simulink library "hdlmdlgenlib"  (R2019a)
settings: Solver=FixedStepDiscrete  StartTime=0.0  StopTime=10.0  FixedStep=1  RelTol=1e-3  EnableMultiTasking=on
libraries: simulink x25, $bdroot x4
settings Model: Creator=The MathWorks, Inc.  LastModifiedBy=The MathWorks, Inc.
settings DataIOCC: LimitDataPoints=on  SaveFormat=Array  ReturnWorkspaceOutputs=off
settings OptimizationCC: ExpressionDepthLimit=2147483647  LifeSpan=inf
settings DebuggingCC: UnderspecifiedInitializationDetection=Classic  MergeDetectMultiDrivingBlocksExec=none  SolverPrmCheckMsg=warning  FcnCallInpInsideContextMsg=warning  AllowSymbolicDim=off  StateNameClashWarn=warning  PregeneratedLibrarySubsystemCodeDiagnostic=none  SFUnexpectedBacktrackingDiag=warning  SFNoUnconditionalDefaultTransitionDiag=warning  SFExecutionAtInitializationDiag=none  ArithmeticOperatorsInVariantConditions=warning
settings HardwareCC: ProdBitPerPointer=32  ProdBitPerSizeT=32  ProdBitPerPtrDiffT=32  ProdLargestAtomicFloat=None  ProdIntDivRoundTo=Undefined  ProdEndianess=Unspecified  ProdWordSize=32  ProdHWDeviceType=32-bit Generic
settings ModelReferenceCC: PropagateSignalLabelsOutOfModel=off
settings SFSimCC: SimUseLocalCustomCode=off
settings RTWCC: RTWUseLocalCustomCode=off
settings CodeAppCC: StateflowObjectComments=on
settings GRTTargetCC: TargetLangStandard=C89/C90 (ANSI)  GeneratePreprocessorConditionals=Disable all  CombineOutputUpdateFcns=off  GRTInterface=on
settings ConfigComp: CovMetricSettings=dw  CovHtmlReporting=on  CovSaveCumulativeToWorkspaceVar=on  CovSaveSingleToWorkspaceVar=on  CovShowResultsExplorer=off  CovExternalEMLEnable=off

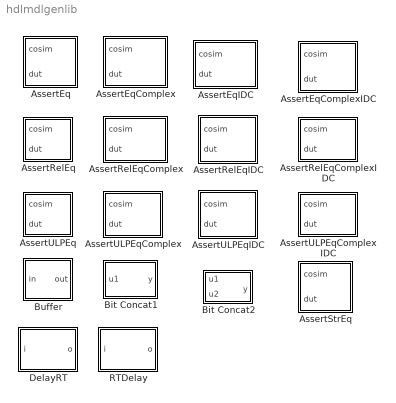
== system hdlmdlgenlib ==
  AssertEq : Subsystem
  AssertEqComplex : Subsystem
  AssertEqComplexIDC : Subsystem
  AssertEqIDC : Subsystem
  AssertRelEq : Subsystem  mask{ToleranceValue=1e-7}
  AssertRelEqComplex : Subsystem  mask{ToleranceValue=1e-7}
  AssertRelEqComplexIDC : Subsystem  mask{ToleranceValue=1e-7}
  AssertRelEqIDC : Subsystem  mask{ToleranceValue=1e-7}
  AssertStrEq : Subsystem  AncestorBlock=hdlmdlgenlib/AssertEq
  AssertULPEq : Subsystem  mask{ToleranceValue=0}
  AssertULPEqComplex : Subsystem  mask{ToleranceValue=0}
  AssertULPEqComplexIDC : Subsystem  mask{ToleranceValue=0}
  AssertULPEqIDC : Subsystem  mask{ToleranceValue=0}
  Bit Concat1 : Subsystem  TreatAsAtomicUnit=on  mask(Bit Concat){}
      mask help: Concatenate the input words.
      mask init:
      | blkname = 'Concat';
      mask Help: helpview([docroot '/toolbox/hdlcoder/ug/hdlcoder_ug.map'],'HDL_bitwise_operator');
      mask Display: disp(blkname);
  Bit Concat2 : Subsystem  TreatAsAtomicUnit=on  mask(Bit Concat){}
      mask help: Concatenate the input words.
      mask init:
      | blkname = 'Concat';
      mask Help: helpview([docroot '/toolbox/hdlcoder/ug/hdlcoder_ug.map'],'HDL_bitwise_operator');
      mask Display: disp(blkname);
  Buffer : Subsystem  mask(Buffer/Wire){}
      mask help: Buffer
  DelayRT : Subsystem
  RTDelay : Subsystem

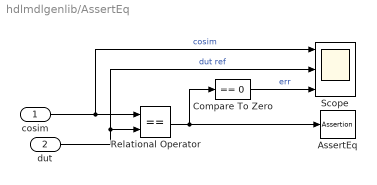
== system hdlmdlgenlib/AssertEq ==
  cosim : Inport
  dut : Inport  Port=2
  AssertEq : Assertion  StopWhenAssertionFail=off
  Compare To Zero : simulink/Logic and Bit Operations/Compare To Zero  relop===  OutDataTypeStr=boolean
  Relational Operator : RelationalOperator  Operator===  OutDataTypeStr=boolean  RndMeth=Nearest
  Scope : Scope  NumInputPorts=3
  wires:
  dut/1 -> Relational Operator/2, Scope/2  "dut ref"
  cosim/1 -> Relational Operator/1, Scope/1  "cosim"
  Relational Operator/1 -> AssertEq/1, Compare To Zero/1
  Compare To Zero/1 -> Scope/3  "err"

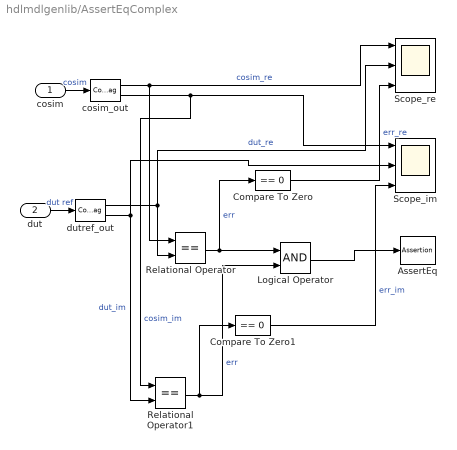
== system hdlmdlgenlib/AssertEqComplex ==
  cosim : Inport
  dut : Inport  Port=2
  AssertEq : Assertion  StopWhenAssertionFail=off
  Compare To Zero : simulink/Logic and Bit Operations/Compare To Zero  relop===  OutDataTypeStr=boolean
  Compare To Zero1 : simulink/Logic and Bit Operations/Compare To Zero  relop===  OutDataTypeStr=boolean
  Logical Operator : Logic  AllPortsSameDT=off  OutDataTypeStr=boolean
  Relational Operator : RelationalOperator  Operator===  OutDataTypeStr=boolean  RndMeth=Nearest
  Relational Operator1 : RelationalOperator  Operator===  OutDataTypeStr=boolean  RndMeth=Nearest
  Scope_im : Scope  NumInputPorts=3
  Scope_re : Scope  NumInputPorts=3
  cosim_out : ComplexToRealImag
  dutref_out : ComplexToRealImag
  wires:
  Relational Operator/1 -> Logical Operator/1, Compare To Zero/1  "err"
  cosim/1 -> cosim_out/1  "cosim"
  dut/1 -> dutref_out/1  "dut ref"
  cosim_out/1 -> Relational Operator/1, Scope_re/1  "cosim_re"
  dutref_out/1 -> Scope_re/2, Relational Operator/2  "dut_re"
  Compare To Zero/1 -> Scope_re/3  "err_re"
  cosim_out/2 -> Relational Operator1/1, Scope_im/1  "cosim_im"
  dutref_out/2 -> Scope_im/2, Relational Operator1/2  "dut_im"
  Compare To Zero1/1 -> Scope_im/3  "err_im"
  Logical Operator/1 -> AssertEq/1
  Relational Operator1/1 -> Logical Operator/2, Compare To Zero1/1  "err"

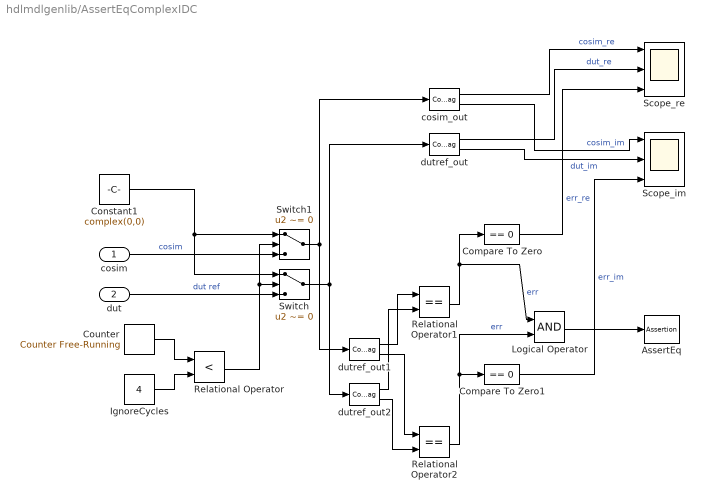
== system hdlmdlgenlib/AssertEqComplexIDC ==
  cosim : Inport
  dut : Inport  Port=2
  AssertEq : Assertion  StopWhenAssertionFail=off
  Compare To Zero : simulink/Logic and Bit Operations/Compare To Zero  relop===  OutDataTypeStr=boolean
  Compare To Zero1 : simulink/Logic and Bit Operations/Compare To Zero  relop===  OutDataTypeStr=boolean
  Constant1 : Constant  Value=complex(0,0)  OutDataTypeStr=Inherit: Inherit via back propagation  SampleTime=-1
  Counter : simulink/Sources/Counter Free-Running  NumBits=32  tsamp=-1
  IgnoreCycles : Constant  Value=4  OutDataTypeStr=Inherit: Inherit via back propagation  SampleTime=-1
  Logical Operator : Logic  AllPortsSameDT=off  OutDataTypeStr=boolean
  Relational Operator : RelationalOperator  Operator=<  OutDataTypeStr=boolean  RndMeth=Nearest
  Relational Operator1 : RelationalOperator  Operator===  OutDataTypeStr=boolean  RndMeth=Nearest
  Relational Operator2 : RelationalOperator  Operator===  OutDataTypeStr=boolean  RndMeth=Nearest
  Scope_im : Scope  NumInputPorts=3
  Scope_re : Scope  NumInputPorts=3
  Switch : Switch  Criteria=u2 ~= 0
  Switch1 : Switch  Criteria=u2 ~= 0
  cosim_out : ComplexToRealImag
  dutref_out : ComplexToRealImag
  dutref_out1 : ComplexToRealImag
  dutref_out2 : ComplexToRealImag
  wires:
  Compare To Zero1/1 -> Scope_im/3  "err_im"
  dutref_out/2 -> Scope_im/2  "dut_im"
  cosim_out/2 -> Scope_im/1  "cosim_im"
  Compare To Zero/1 -> Scope_re/3  "err_re"
  dutref_out/1 -> Scope_re/2  "dut_re"
  cosim_out/1 -> Scope_re/1  "cosim_re"
  Relational Operator1/1 -> Logical Operator/1, Compare To Zero/1  "err"
  Switch1/1 -> dutref_out1/1, cosim_out/1
  Switch/1 -> dutref_out2/1, dutref_out/1
  Constant1/1 -> Switch1/1, Switch/1
  Relational Operator/1 -> Switch1/2, Switch/2
  cosim/1 -> Switch1/3  "cosim"
  dut/1 -> Switch/3  "dut ref"
  Counter/1 -> Relational Operator/1
  IgnoreCycles/1 -> Relational Operator/2
  Logical Operator/1 -> AssertEq/1
  dutref_out1/1 -> Relational Operator1/1
  dutref_out2/1 -> Relational Operator1/2
  dutref_out2/2 -> Relational Operator2/2
  dutref_out1/2 -> Relational Operator2/1
  Relational Operator2/1 -> Logical Operator/2, Compare To Zero1/1  "err"

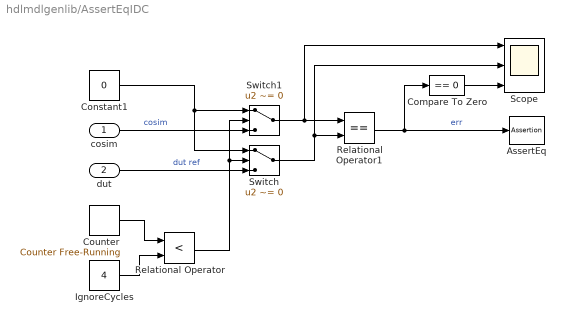
== system hdlmdlgenlib/AssertEqIDC ==
  cosim : Inport
  dut : Inport  Port=2
  AssertEq : Assertion  StopWhenAssertionFail=off
  Compare To Zero : simulink/Logic and Bit Operations/Compare To Zero  relop===  OutDataTypeStr=boolean
  Constant1 : Constant  Value=0  OutDataTypeStr=Inherit: Inherit via back propagation  SampleTime=-1
  Counter : simulink/Sources/Counter Free-Running  NumBits=32  tsamp=-1
  IgnoreCycles : Constant  Value=4  OutDataTypeStr=Inherit: Inherit via back propagation  SampleTime=-1
  Relational Operator : RelationalOperator  Operator=<  OutDataTypeStr=boolean  RndMeth=Nearest
  Relational Operator1 : RelationalOperator  Operator===  OutDataTypeStr=boolean  RndMeth=Nearest
  Scope : Scope  NumInputPorts=3
  Switch : Switch  Criteria=u2 ~= 0
  Switch1 : Switch  Criteria=u2 ~= 0
  wires:
  IgnoreCycles/1 -> Relational Operator/2
  Counter/1 -> Relational Operator/1
  dut/1 -> Switch/3  "dut ref"
  cosim/1 -> Switch1/3  "cosim"
  Relational Operator/1 -> Switch1/2, Switch/2
  Constant1/1 -> Switch1/1, Switch/1
  Switch/1 -> Relational Operator1/2, Scope/2
  Switch1/1 -> Relational Operator1/1, Scope/1
  Relational Operator1/1 -> AssertEq/1, Compare To Zero/1  "err"
  Compare To Zero/1 -> Scope/3

== system hdlmdlgenlib/AssertRelEq ==
  cosim : Inport
  dut : Inport  Port=2
  AssertEq : Assertion  StopWhenAssertionFail=off
  Compare To Zero : simulink/Logic and Bit Operations/Compare To Zero  relop===  OutDataTypeStr=boolean
  RelErrCheck : Subsystem
  Scope : Scope  NumInputPorts=3
  wires:
  Compare To Zero/1 -> Scope/3  "err"
  RelErrCheck/1(Out1) -> Compare To Zero/1, AssertEq/1
  cosim/1 -> RelErrCheck/1(In1), Scope/1  "cosim"
  dut/1 -> RelErrCheck/2(In2), Scope/2  "dut ref"

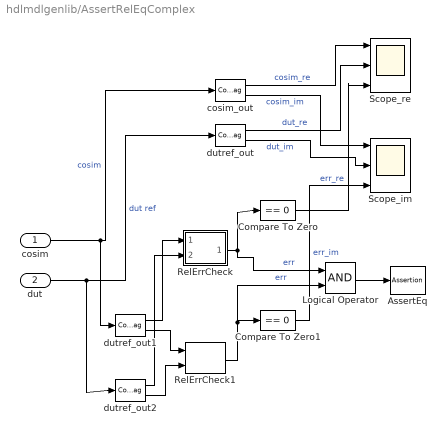
== system hdlmdlgenlib/AssertRelEqComplex ==
  cosim : Inport
  dut : Inport  Port=2
  AssertEq : Assertion  StopWhenAssertionFail=off
  Compare To Zero : simulink/Logic and Bit Operations/Compare To Zero  relop===  OutDataTypeStr=boolean
  Compare To Zero1 : simulink/Logic and Bit Operations/Compare To Zero  relop===  OutDataTypeStr=boolean
  Logical Operator : Logic  AllPortsSameDT=off  OutDataTypeStr=boolean
  RelErrCheck : Subsystem
  RelErrCheck1 : $bdroot/AssertRelEqComplex/RelErrCheck  SystemSampleTime=-1
  Scope_im : Scope  NumInputPorts=3
  Scope_re : Scope  NumInputPorts=3
  cosim_out : ComplexToRealImag
  dutref_out : ComplexToRealImag
  dutref_out1 : ComplexToRealImag
  dutref_out2 : ComplexToRealImag
  wires:
  Compare To Zero1/1 -> Scope_im/3  "err_im"
  dutref_out/2 -> Scope_im/2  "dut_im"
  cosim_out/2 -> Scope_im/1  "cosim_im"
  Compare To Zero/1 -> Scope_re/3  "err_re"
  dutref_out/1 -> Scope_re/2  "dut_re"
  cosim_out/1 -> Scope_re/1  "cosim_re"
  dut/1 -> dutref_out2/1, dutref_out/1  "dut ref"
  cosim/1 -> cosim_out/1, dutref_out1/1  "cosim"
  RelErrCheck/1(Out1) -> Logical Operator/1, Compare To Zero/1  "err"
  Logical Operator/1 -> AssertEq/1
  dutref_out1/1 -> RelErrCheck/1(In1)
  dutref_out2/1 -> RelErrCheck/2(In2)
  dutref_out2/2 -> RelErrCheck1/2
  dutref_out1/2 -> RelErrCheck1/1
  RelErrCheck1/1 -> Logical Operator/2, Compare To Zero1/1  "err"

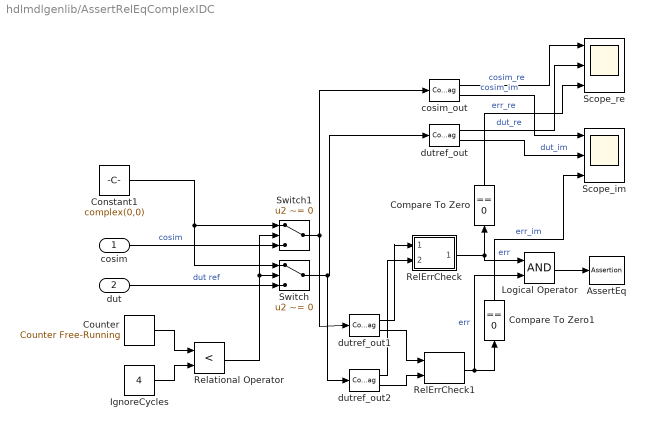
== system hdlmdlgenlib/AssertRelEqComplexIDC ==
  cosim : Inport
  dut : Inport  Port=2
  AssertEq : Assertion  StopWhenAssertionFail=off
  Compare To Zero : simulink/Logic and Bit Operations/Compare To Zero  relop===  OutDataTypeStr=boolean
  Compare To Zero1 : simulink/Logic and Bit Operations/Compare To Zero  relop===  OutDataTypeStr=boolean
  Constant1 : Constant  Value=complex(0,0)  OutDataTypeStr=Inherit: Inherit via back propagation  SampleTime=-1
  Counter : simulink/Sources/Counter Free-Running  NumBits=32  tsamp=-1
  IgnoreCycles : Constant  Value=4  OutDataTypeStr=Inherit: Inherit via back propagation  SampleTime=-1
  Logical Operator : Logic  AllPortsSameDT=off  OutDataTypeStr=boolean
  RelErrCheck : Subsystem
  RelErrCheck1 : $bdroot/AssertRelEqComplexIDC/RelErrCheck  SystemSampleTime=-1
  Relational Operator : RelationalOperator  Operator=<  OutDataTypeStr=boolean  RndMeth=Nearest
  Scope_im : Scope  NumInputPorts=3
  Scope_re : Scope  NumInputPorts=3
  Switch : Switch  Criteria=u2 ~= 0
  Switch1 : Switch  Criteria=u2 ~= 0
  cosim_out : ComplexToRealImag
  dutref_out : ComplexToRealImag
  dutref_out1 : ComplexToRealImag
  dutref_out2 : ComplexToRealImag
  wires:
  IgnoreCycles/1 -> Relational Operator/2
  Counter/1 -> Relational Operator/1
  dut/1 -> Switch/3  "dut ref"
  cosim/1 -> Switch1/3  "cosim"
  Relational Operator/1 -> Switch/2, Switch1/2
  Constant1/1 -> Switch/1, Switch1/1
  Switch/1 -> dutref_out2/1, dutref_out/1
  Switch1/1 -> cosim_out/1, dutref_out1/1
  RelErrCheck/1(Out1) -> Logical Operator/1, Compare To Zero/1  "err"
  cosim_out/1 -> Scope_re/1  "cosim_re"
  dutref_out/1 -> Scope_re/2  "dut_re"
  Compare To Zero/1 -> Scope_re/3  "err_re"
  cosim_out/2 -> Scope_im/1  "cosim_im"
  dutref_out/2 -> Scope_im/2  "dut_im"
  Compare To Zero1/1 -> Scope_im/3  "err_im"
  Logical Operator/1 -> AssertEq/1
  dutref_out1/1 -> RelErrCheck/1(In1)
  RelErrCheck1/1 -> Compare To Zero1/1, Logical Operator/2  "err"
  dutref_out2/1 -> RelErrCheck/2(In2)
  dutref_out1/2 -> RelErrCheck1/1
  dutref_out2/2 -> RelErrCheck1/2

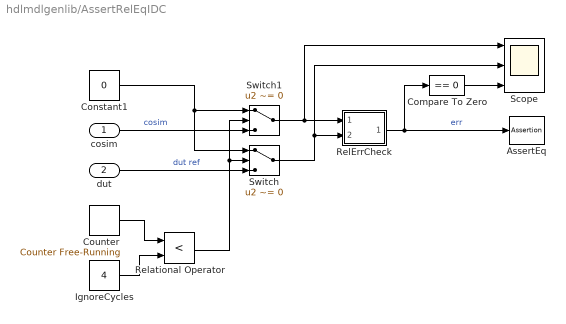
== system hdlmdlgenlib/AssertRelEqIDC ==
  cosim : Inport
  dut : Inport  Port=2
  AssertEq : Assertion  StopWhenAssertionFail=off
  Compare To Zero : simulink/Logic and Bit Operations/Compare To Zero  relop===  OutDataTypeStr=boolean
  Constant1 : Constant  Value=0  OutDataTypeStr=Inherit: Inherit via back propagation  SampleTime=-1
  Counter : simulink/Sources/Counter Free-Running  NumBits=32  tsamp=-1
  IgnoreCycles : Constant  Value=4  OutDataTypeStr=Inherit: Inherit via back propagation  SampleTime=-1
  RelErrCheck : Subsystem
  Relational Operator : RelationalOperator  Operator=<  OutDataTypeStr=boolean  RndMeth=Nearest
  Scope : Scope  NumInputPorts=3
  Switch : Switch  Criteria=u2 ~= 0
  Switch1 : Switch  Criteria=u2 ~= 0
  wires:
  Compare To Zero/1 -> Scope/3
  RelErrCheck/1(Out1) -> Compare To Zero/1, AssertEq/1  "err"
  Switch1/1 -> RelErrCheck/1(In1), Scope/1
  Switch/1 -> RelErrCheck/2(In2), Scope/2
  Constant1/1 -> Switch/1, Switch1/1
  Relational Operator/1 -> Switch/2, Switch1/2
  cosim/1 -> Switch1/3  "cosim"
  dut/1 -> Switch/3  "dut ref"
  Counter/1 -> Relational Operator/1
  IgnoreCycles/1 -> Relational Operator/2

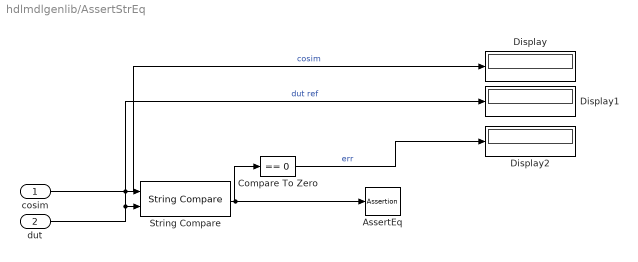
== system hdlmdlgenlib/AssertStrEq ==
  cosim : Inport
  dut : Inport  Port=2
  AssertEq : Assertion  StopWhenAssertionFail=off
  Compare To Zero : simulink/Logic and Bit Operations/Compare To Zero  relop===  OutDataTypeStr=boolean
  Display : Display
  Display1 : Display
  Display2 : Display
  String Compare : StringCompare
  wires:
  dut/1 -> Display1/1, String Compare/2  "dut ref"
  cosim/1 -> Display/1, String Compare/1  "cosim"
  String Compare/1 -> Compare To Zero/1, AssertEq/1
  Compare To Zero/1 -> Display2/1  "err"

== system hdlmdlgenlib/AssertULPEq ==
  cosim : Inport
  dut : Inport  Port=2
  AssertEq : Assertion  StopWhenAssertionFail=off
  Compare To Zero : simulink/Logic and Bit Operations/Compare To Zero  relop===  OutDataTypeStr=boolean
  Scope : Scope  NumInputPorts=3
  ULPChecker : Subsystem
  wires:
  Compare To Zero/1 -> Scope/3  "err"
  ULPChecker/1(Out1) -> Compare To Zero/1, AssertEq/1
  cosim/1 -> ULPChecker/1(In1), Scope/1  "cosim"
  dut/1 -> ULPChecker/2(In2), Scope/2  "dut ref"

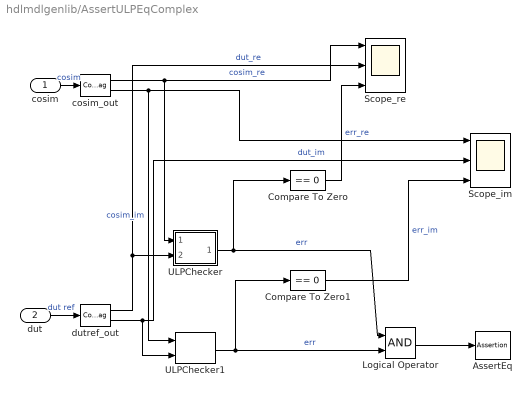
== system hdlmdlgenlib/AssertULPEqComplex ==
  cosim : Inport
  dut : Inport  Port=2
  AssertEq : Assertion  StopWhenAssertionFail=off
  Compare To Zero : simulink/Logic and Bit Operations/Compare To Zero  relop===  OutDataTypeStr=boolean
  Compare To Zero1 : simulink/Logic and Bit Operations/Compare To Zero  relop===  OutDataTypeStr=boolean
  Logical Operator : Logic  AllPortsSameDT=off  OutDataTypeStr=boolean
  Scope_im : Scope  NumInputPorts=3
  Scope_re : Scope  NumInputPorts=3
  ULPChecker : Subsystem
  ULPChecker1 : $bdroot/AssertULPEqComplex/ULPChecker  SystemSampleTime=-1
  cosim_out : ComplexToRealImag
  dutref_out : ComplexToRealImag
  wires:
  ULPChecker/1(Out1) -> Logical Operator/1, Compare To Zero/1  "err"
  cosim/1 -> cosim_out/1  "cosim"
  dut/1 -> dutref_out/1  "dut ref"
  cosim_out/1 -> ULPChecker/1(In1), Scope_re/1  "cosim_re"
  dutref_out/1 -> ULPChecker/2(In2), Scope_re/2  "dut_re"
  Compare To Zero/1 -> Scope_re/3  "err_re"
  cosim_out/2 -> ULPChecker1/1, Scope_im/1  "cosim_im"
  dutref_out/2 -> ULPChecker1/2, Scope_im/2  "dut_im"
  Compare To Zero1/1 -> Scope_im/3  "err_im"
  ULPChecker1/1 -> Compare To Zero1/1, Logical Operator/2  "err"
  Logical Operator/1 -> AssertEq/1

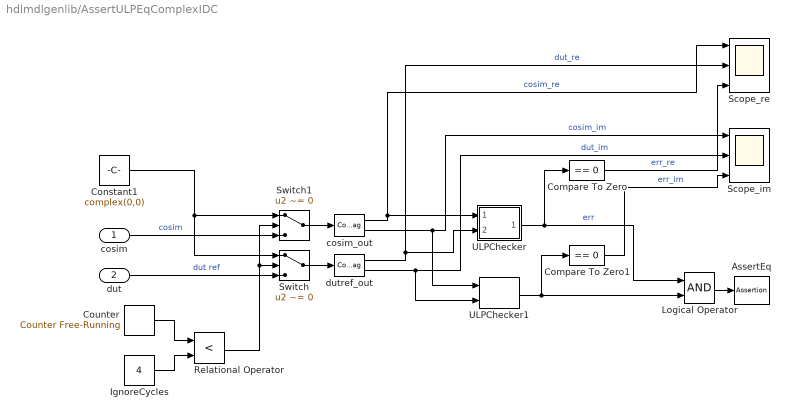
== system hdlmdlgenlib/AssertULPEqComplexIDC ==
  cosim : Inport
  dut : Inport  Port=2
  AssertEq : Assertion  StopWhenAssertionFail=off
  Compare To Zero : simulink/Logic and Bit Operations/Compare To Zero  relop===  OutDataTypeStr=boolean
  Compare To Zero1 : simulink/Logic and Bit Operations/Compare To Zero  relop===  OutDataTypeStr=boolean
  Constant1 : Constant  Value=complex(0,0)  OutDataTypeStr=Inherit: Inherit via back propagation  SampleTime=-1
  Counter : simulink/Sources/Counter Free-Running  NumBits=32  tsamp=-1
  IgnoreCycles : Constant  Value=4  OutDataTypeStr=Inherit: Inherit via back propagation  SampleTime=-1
  Logical Operator : Logic  AllPortsSameDT=off  OutDataTypeStr=boolean
  Relational Operator : RelationalOperator  Operator=<  OutDataTypeStr=boolean  RndMeth=Nearest
  Scope_im : Scope  NumInputPorts=3
  Scope_re : Scope  NumInputPorts=3
  Switch : Switch  Criteria=u2 ~= 0
  Switch1 : Switch  Criteria=u2 ~= 0
  ULPChecker : Subsystem
  ULPChecker1 : $bdroot/AssertULPEqComplexIDC/ULPChecker  SystemSampleTime=-1
  cosim_out : ComplexToRealImag
  dutref_out : ComplexToRealImag
  wires:
  IgnoreCycles/1 -> Relational Operator/2
  Counter/1 -> Relational Operator/1
  dut/1 -> Switch/3  "dut ref"
  cosim/1 -> Switch1/3  "cosim"
  Relational Operator/1 -> Switch/2, Switch1/2
  Constant1/1 -> Switch/1, Switch1/1
  Switch/1 -> dutref_out/1
  Switch1/1 -> cosim_out/1
  ULPChecker/1(Out1) -> Logical Operator/1, Compare To Zero/1  "err"
  cosim_out/1 -> ULPChecker/1(In1), Scope_re/1  "cosim_re"
  dutref_out/1 -> ULPChecker/2(In2), Scope_re/2  "dut_re"
  Compare To Zero/1 -> Scope_re/3  "err_re"
  cosim_out/2 -> ULPChecker1/1, Scope_im/1  "cosim_im"
  dutref_out/2 -> ULPChecker1/2, Scope_im/2  "dut_im"
  Compare To Zero1/1 -> Scope_im/3  "err_im"
  Logical Operator/1 -> AssertEq/1
  ULPChecker1/1 -> Compare To Zero1/1, Logical Operator/2

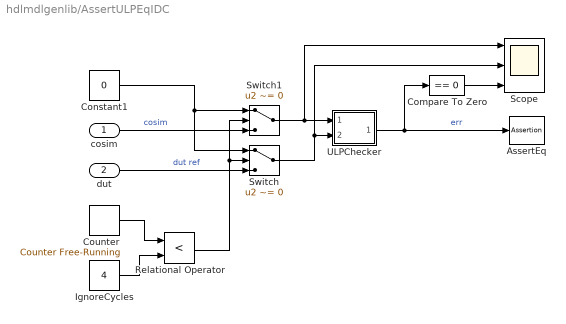
== system hdlmdlgenlib/AssertULPEqIDC ==
  cosim : Inport
  dut : Inport  Port=2
  AssertEq : Assertion  StopWhenAssertionFail=off
  Compare To Zero : simulink/Logic and Bit Operations/Compare To Zero  relop===  OutDataTypeStr=boolean
  Constant1 : Constant  Value=0  OutDataTypeStr=Inherit: Inherit via back propagation  SampleTime=-1
  Counter : simulink/Sources/Counter Free-Running  NumBits=32  tsamp=-1
  IgnoreCycles : Constant  Value=4  OutDataTypeStr=Inherit: Inherit via back propagation  SampleTime=-1
  Relational Operator : RelationalOperator  Operator=<  OutDataTypeStr=boolean  RndMeth=Nearest
  Scope : Scope  NumInputPorts=3
  Switch : Switch  Criteria=u2 ~= 0
  Switch1 : Switch  Criteria=u2 ~= 0
  ULPChecker : Subsystem
  wires:
  Compare To Zero/1 -> Scope/3
  ULPChecker/1(Out1) -> Compare To Zero/1, AssertEq/1  "err"
  Switch1/1 -> ULPChecker/1(In1), Scope/1
  Switch/1 -> ULPChecker/2(In2), Scope/2
  Constant1/1 -> Switch/1, Switch1/1
  Relational Operator/1 -> Switch/2, Switch1/2
  cosim/1 -> Switch1/3  "cosim"
  dut/1 -> Switch/3  "dut ref"
  Counter/1 -> Relational Operator/1
  IgnoreCycles/1 -> Relational Operator/2

== system hdlmdlgenlib/Bit Concat1 ==
  u1 : Inport
  bit_concat_unary : MATLAB Function  TreatAsAtomicUnit=on
  y : Outport
  wires:
  bit_concat_unary/1(y) -> y/1
  u1/1 -> bit_concat_unary/1(u)

== system hdlmdlgenlib/Bit Concat2 ==
  u1 : Inport
  u2 : Inport  Port=2
  bit_concat : MATLAB Function  TreatAsAtomicUnit=on
  y : Outport
  wires:
  u2/1 -> bit_concat/2(u2)
  u1/1 -> bit_concat/1(u1)
  bit_concat/1(y) -> y/1

== system hdlmdlgenlib/Buffer ==
  in : Inport
  out : Outport
  wires:
  in/1 -> out/1

== system hdlmdlgenlib/DelayRT ==
  i : Inport
  Delay : Delay  DelayLength=1  InitialCondition=0
  RT : RateTransition  OutPortSampleTimeOpt=Multiple of input port sample time  OutPortSampleTimeMultiple=2
  o : Outport
  wires:
  i/1 -> Delay/1  "cosim"
  Delay/1 -> RT/1
  RT/1 -> o/1

== system hdlmdlgenlib/RTDelay ==
  i : Inport
  Delay : Delay  DelayLength=1  InitialCondition=0
  RT : RateTransition  OutPortSampleTimeOpt=Multiple of input port sample time  OutPortSampleTimeMultiple=2
  o : Outport
  wires:
  RT/1 -> Delay/1
  i/1 -> RT/1  "cosim"
  Delay/1 -> o/1

== system hdlmdlgenlib/AssertRelEq/RelErrCheck ==
  In1 : Inport
  In2 : Inport  Port=2
  "RelativeErrorCheck " : MATLAB Function  TreatAsAtomicUnit=on
  Out1 : Outport
  wires:
  "RelativeErrorCheck "/1(y) -> Out1/1
  In1/1 -> "RelativeErrorCheck "/1(P)
  In2/1 -> "RelativeErrorCheck "/2(R)

== system hdlmdlgenlib/AssertRelEqComplex/RelErrCheck ==
  In1 : Inport
  In2 : Inport  Port=2
  "RelativeErrorCheck " : MATLAB Function  TreatAsAtomicUnit=on
  Out1 : Outport
  wires:
  In2/1 -> "RelativeErrorCheck "/2(R)
  In1/1 -> "RelativeErrorCheck "/1(P)
  "RelativeErrorCheck "/1(y) -> Out1/1

== system hdlmdlgenlib/AssertRelEqComplexIDC/RelErrCheck ==
  In1 : Inport
  In2 : Inport  Port=2
  "RelativeErrorCheck " : MATLAB Function  TreatAsAtomicUnit=on
  Out1 : Outport
  wires:
  In2/1 -> "RelativeErrorCheck "/2(R)
  In1/1 -> "RelativeErrorCheck "/1(P)
  "RelativeErrorCheck "/1(y) -> Out1/1

== system hdlmdlgenlib/AssertRelEqIDC/RelErrCheck ==
  In1 : Inport
  In2 : Inport  Port=2
  "RelativeErrorCheck " : MATLAB Function  TreatAsAtomicUnit=on
  Out1 : Outport
  wires:
  In2/1 -> "RelativeErrorCheck "/2(R)
  In1/1 -> "RelativeErrorCheck "/1(P)
  "RelativeErrorCheck "/1(y) -> Out1/1

== system hdlmdlgenlib/AssertULPEq/ULPChecker ==
  In1 : Inport
  In2 : Inport  Port=2
  "ULPErrorCheck " : MATLAB Function  TreatAsAtomicUnit=on
  Out1 : Outport
  wires:
  In2/1 -> "ULPErrorCheck "/2(R)
  In1/1 -> "ULPErrorCheck "/1(P)
  "ULPErrorCheck "/1(y) -> Out1/1

== system hdlmdlgenlib/AssertULPEqComplex/ULPChecker ==
  In1 : Inport
  In2 : Inport  Port=2
  ULPErrorCheck : MATLAB Function  TreatAsAtomicUnit=on
  Out1 : Outport
  wires:
  ULPErrorCheck/1(y) -> Out1/1
  In1/1 -> ULPErrorCheck/1(P)
  In2/1 -> ULPErrorCheck/2(R)

== system hdlmdlgenlib/AssertULPEqComplexIDC/ULPChecker ==
  In1 : Inport
  In2 : Inport  Port=2
  "ULPErrorCheck " : MATLAB Function  TreatAsAtomicUnit=on
  Out1 : Outport
  wires:
  "ULPErrorCheck "/1(y) -> Out1/1
  In1/1 -> "ULPErrorCheck "/1(P)
  In2/1 -> "ULPErrorCheck "/2(R)

== system hdlmdlgenlib/AssertULPEqIDC/ULPChecker ==
  In1 : Inport
  In2 : Inport  Port=2
  "ULPErrorCheck " : MATLAB Function  TreatAsAtomicUnit=on
  Out1 : Outport
  wires:
  "ULPErrorCheck "/1(y) -> Out1/1
  In1/1 -> "ULPErrorCheck "/1(P)
  In2/1 -> "ULPErrorCheck "/2(R)

== matlab function hdlmdlgenlib/Bit Concat1/bit_concat_unary ==
  data: u input; y output
function y = fcn(u)
%#codegen

y = bitconcat(cast_to_fi(u));

end

== matlab function hdlmdlgenlib/AssertULPEqComplex/ULPChecker/ULPErrorCheck ==
  data: P input; y output; R input; ToleranceValue parameter uint32
function y = ulpErrCheck(P,R, ToleranceValue)
ulp = ToleranceValue;
sz = numel(P);
assert(sz == numel(R), 'Inputs P and R have different sizes.');
y = false(1, sz);

for ii=1:sz
    if isa(P(ii), 'single')
        P_fpt = fi(typecast(single(P(ii)),'int32'),1,32,0);
        R_fpt = fi(typecast(single(R(ii)),'int32'),1,32,0);
        tmp = bitset(P_fpt, 32, 1);
        if (P_fpt < 0)
            % lexographic two's complement ordering
            P_fpt = fi(tmp - P_fpt, 1, 33, 0);
        else
            P_fpt = fi(P_fpt, 1, 33, 0);
        end
        if (R_fpt < 0)
            % lexographic two's complement ordering
            R_fpt = fi(tmp - R_fpt, 1, 33, 0);
        else
            R_fpt = fi(R_fpt, 1, 33, 0);
        end
        error = abs(P_fpt - R_fpt);
    elseif isa(P(ii), 'double')
        P_fpt = fi(typecast(double(P(ii)),'int64'),1,64,0);
        R_fpt = fi(typecast(double(R(ii)),'int64'),1,64,0);
        tmp = bitset(P_fpt, 64, 1);
        if (P_fpt < 0)
            % lexographic two's complement ordering
            P_fpt = fi(tmp - P_fpt, 1, 65, 0);
        else
            P_fpt = fi(P_fpt, 1, 65, 0);
        end
        if (R_fpt < 0)
            % lexographic two's complement ordering
            R_fpt = fi(tmp - R_fpt, 1, 65, 0);
        else
            R_fpt = fi(R_fpt, 1, 65, 0);
        end
        error = abs(P_fpt - R_fpt);
    else
        assert(0, 'Input data type is not floating point.');
    end
    
    if(error > ulp)
        y(ii) = false;
    else
        y(ii) = true;
    end
end

== matlab function hdlmdlgenlib/AssertULPEqIDC/ULPChecker/ULPErrorCheck  ==
  data: P input; y output; R input; ToleranceValue parameter uint32
function y = ulpErrCheck(P,R, ToleranceValue)
ulp = ToleranceValue;
sz = numel(P);
assert(sz == numel(R), 'Inputs P and R have different sizes.');
y = false(1, sz);

for ii=1:sz
    if isa(P(ii), 'single')
        P_fpt = fi(typecast(single(P(ii)),'int32'),1,32,0);
        R_fpt = fi(typecast(single(R(ii)),'int32'),1,32,0);
        tmp = bitset(P_fpt, 32, 1);
        if (P_fpt < 0)
            % lexographic two's complement ordering
            P_fpt = fi(tmp - P_fpt, 1, 33, 0);
        else
            P_fpt = fi(P_fpt, 1, 33, 0);
        end
        if (R_fpt < 0)
            % lexographic two's complement ordering
            R_fpt = fi(tmp - R_fpt, 1, 33, 0);
        else
            R_fpt = fi(R_fpt, 1, 33, 0);
        end
        error = abs(P_fpt - R_fpt);
    elseif isa(P(ii), 'double')
        P_fpt = fi(typecast(double(P(ii)),'int64'),1,64,0);
        R_fpt = fi(typecast(double(R(ii)),'int64'),1,64,0);
        tmp = bitset(P_fpt, 64, 1);
        if (P_fpt < 0)
            % lexographic two's complement ordering
            P_fpt = fi(tmp - P_fpt, 1, 65, 0);
        else
            P_fpt = fi(P_fpt, 1, 65, 0);
        end
        if (R_fpt < 0)
            % lexographic two's complement ordering
            R_fpt = fi(tmp - R_fpt, 1, 65, 0);
        else
            R_fpt = fi(R_fpt, 1, 65, 0);
        end
        error = abs(P_fpt - R_fpt);
    else
        assert(0, 'Input data type is not floating point.');
    end
    
    if(error > ulp)
        y(ii) = false;
    else
        y(ii) = true;
    end
end

== matlab function hdlmdlgenlib/AssertULPEqComplexIDC/ULPChecker/ULPErrorCheck  ==
  data: P input; y output; R input; ToleranceValue parameter uint32
function y = ulpErrCheck(P,R, ToleranceValue)
ulp = ToleranceValue;
sz = numel(P);
assert(sz == numel(R), 'Inputs P and R have different sizes.');
y = false(1, sz);

for ii=1:sz
    if isa(P(ii), 'single')
        P_fpt = fi(typecast(single(P(ii)),'int32'),1,32,0);
        R_fpt = fi(typecast(single(R(ii)),'int32'),1,32,0);
        tmp = bitset(P_fpt, 32, 1);
        if (P_fpt < 0)
            % lexographic two's complement ordering
            P_fpt = fi(tmp - P_fpt, 1, 33, 0);
        else
            P_fpt = fi(P_fpt, 1, 33, 0);
        end
        if (R_fpt < 0)
            % lexographic two's complement ordering
            R_fpt = fi(tmp - R_fpt, 1, 33, 0);
        else
            R_fpt = fi(R_fpt, 1, 33, 0);
        end
        error = abs(P_fpt - R_fpt);
    elseif isa(P(ii), 'double')
        P_fpt = fi(typecast(double(P(ii)),'int64'),1,64,0);
        R_fpt = fi(typecast(double(R(ii)),'int64'),1,64,0);
        tmp = bitset(P_fpt, 64, 1);
        if (P_fpt < 0)
            % lexographic two's complement ordering
            P_fpt = fi(tmp - P_fpt, 1, 65, 0);
        else
            P_fpt = fi(P_fpt, 1, 65, 0);
        end
        if (R_fpt < 0)
            % lexographic two's complement ordering
            R_fpt = fi(tmp - R_fpt, 1, 65, 0);
        else
            R_fpt = fi(R_fpt, 1, 65, 0);
        end
        error = abs(P_fpt - R_fpt);
    else
        assert(0, 'Input data type is not floating point.');
    end
    
    if(error > ulp)
        y(ii) = false;
    else
        y(ii) = true;
    end
end

== matlab function hdlmdlgenlib/Bit Concat2/bit_concat ==
  data: u1 input; y output; u2 input
function y = fcn(u1, u2)
%#codegen

y = bitconcat(cast_to_fi(u1), cast_to_fi(u2));

end

== matlab function hdlmdlgenlib/AssertRelEqComplex/RelErrCheck/RelativeErrorCheck  ==
  data: P input; y output; R input; ToleranceValue parameter double
% Check if the relative error of R with respect to P is below
% ToleranceValue
% P, R are floating-point
function y = relErrCheck(P,R, ToleranceValue)
    tol = ToleranceValue;
    sz = numel(P);
    assert(sz == numel(R), 'Inputs P and R have different sizes.');
    y = false(1, sz);

    for ii=1:sz
        if (isnan(P(ii)) || isnan(R(ii)))
            if (isnan(P(ii)) && isnan(R(ii)))
                y(ii) = true;
            end
        elseif (isinf(P(ii)) || isinf(R(ii)))
            y(ii) = (P(ii) == R(ii));
        elseif (P(ii) == 0)
            y(ii) = (R(ii) == 0);
        else
            absdiff = abs(P(ii) - R(ii));
            relerr = absdiff/abs(P(ii));
            y(ii) = (relerr <= tol);
        end
    end
end

== matlab function hdlmdlgenlib/AssertRelEq/RelErrCheck/RelativeErrorCheck  ==
  data: P input; y output; R input; ToleranceValue parameter double
% Check if the relative error of R with respect to P is below
% ToleranceValue
% P, R are floating-point
function y = relErrCheck(P,R, ToleranceValue)
    tol = ToleranceValue;
    sz = numel(P);
    assert(sz == numel(R), 'Inputs P and R have different sizes.');
    y = false(1, sz);

    for ii=1:sz
        if (isnan(P(ii)) || isnan(R(ii)))
            if (isnan(P(ii)) && isnan(R(ii)))
                y(ii) = true;
            end
        elseif (isinf(P(ii)) || isinf(R(ii)))
            y(ii) = (P(ii) == R(ii));
        elseif (P(ii) == 0)
            y(ii) = (R(ii) == 0);
        else
            absdiff = abs(P(ii) - R(ii));
            relerr = absdiff/abs(P(ii));
            y(ii) = (relerr <= tol);
        end
    end
end

== matlab function hdlmdlgenlib/AssertRelEqIDC/RelErrCheck/RelativeErrorCheck  ==
  data: P input; y output; R input; ToleranceValue parameter double
% Check if the relative error of R with respect to P is below
% ToleranceValue
% P, R are floating-point
function y = relErrCheck(P,R, ToleranceValue)
    tol = ToleranceValue;
    sz = numel(P);
    assert(sz == numel(R), 'Inputs P and R have different sizes.');
    y = false(1, sz);

    for ii=1:sz
        if (isnan(P(ii)) || isnan(R(ii)))
            if (isnan(P(ii)) && isnan(R(ii)))
                y(ii) = true;
            end
        elseif (isinf(P(ii)) || isinf(R(ii)))
            y(ii) = (P(ii) == R(ii));
        elseif (P(ii) == 0)
            y(ii) = (R(ii) == 0);
        else
            absdiff = abs(P(ii) - R(ii));
            relerr = absdiff/abs(P(ii));
            y(ii) = (relerr <= tol);
        end
    end
end

== matlab function hdlmdlgenlib/AssertRelEqComplexIDC/RelErrCheck/RelativeErrorCheck  ==
  data: P input; y output; R input; ToleranceValue parameter double
% Check if the relative error of R with respect to P is below
% ToleranceValue
% P, R are floating-point
function y = relErrCheck(P,R, ToleranceValue)
    tol = ToleranceValue;
    sz = numel(P);
    assert(sz == numel(R), 'Inputs P and R have different sizes.');
    y = false(1, sz);

    for ii=1:sz
        if (isnan(P(ii)) || isnan(R(ii)))
            if (isnan(P(ii)) && isnan(R(ii)))
                y(ii) = true;
            end
        elseif (isinf(P(ii)) || isinf(R(ii)))
            y(ii) = (P(ii) == R(ii));
        elseif (P(ii) == 0)
            y(ii) = (R(ii) == 0);
        else
            absdiff = abs(P(ii) - R(ii));
            relerr = absdiff/abs(P(ii));
            y(ii) = (relerr <= tol);
        end
    end
end

== matlab function hdlmdlgenlib/AssertULPEq/ULPChecker/ULPErrorCheck  ==
  data: P input; y output; R input; ToleranceValue parameter uint32
function y = ulpErrCheck(P,R, ToleranceValue)
ulp = ToleranceValue;
sz = numel(P);
assert(sz == numel(R), 'Inputs P and R have different sizes.');
y = false(1, sz);

for ii=1:sz
    if isa(P(ii), 'single')
        P_fpt = fi(typecast(single(P(ii)),'int32'),1,32,0);
        R_fpt = fi(typecast(single(R(ii)),'int32'),1,32,0);
        tmp = bitset(P_fpt, 32, 1);
        if (P_fpt < 0)
            % lexographic two's complement ordering
            P_fpt = fi(tmp - P_fpt, 1, 33, 0);
        else
            P_fpt = fi(P_fpt, 1, 33, 0);
        end
        if (R_fpt < 0)
            % lexographic two's complement ordering
            R_fpt = fi(tmp - R_fpt, 1, 33, 0);
        else
            R_fpt = fi(R_fpt, 1, 33, 0);
        end
        error = abs(P_fpt - R_fpt);
    elseif isa(P(ii), 'double')
        P_fpt = fi(typecast(double(P(ii)),'int64'),1,64,0);
        R_fpt = fi(typecast(double(R(ii)),'int64'),1,64,0);
        tmp = bitset(P_fpt, 64, 1);
        if (P_fpt < 0)
            % lexographic two's complement ordering
            P_fpt = fi(tmp - P_fpt, 1, 65, 0);
        else
            P_fpt = fi(P_fpt, 1, 65, 0);
        end
        if (R_fpt < 0)
            % lexographic two's complement ordering
            R_fpt = fi(tmp - R_fpt, 1, 65, 0);
        else
            R_fpt = fi(R_fpt, 1, 65, 0);
        end
        error = abs(P_fpt - R_fpt);
    else
        assert(0, 'Input data type is not floating point.');
    end
    
    if(error > ulp)
        y(ii) = false;
    else
        y(ii) = true;
    end
end
